simulink model "SWC_FDC_type"  (R2021b)
settings: Solver=FixedStepDiscrete  StartTime=0.0  StopTime=10.0  FixedStep=0.001  RelTol=1e-3
values from neighbouring files (symbols this model uses):
  C_TASK_5MS_S = (	C_TICK_TIME_S      	)    [vcu_local_hdr.m]
  DID_VCUKey = uint16(0x0202)    [vcu_local_hdr.m]
  DID_XWD = uint16(513)    [vcu_local_hdr.m]
  DIDLen_APPPedalZP = uint16(3)    [vcu_local_hdr.m]
  DIDLen_APSFunConfig = uint16(16)    [vcu_local_hdr.m]
  DIDLen_AutoLock = uint16(1)    [vcu_local_hdr.m]
  DIDLen_AutoWipHSpdEN = uint16(1)    [vcu_local_hdr.m]
  DIDLen_DKCKey = uint16(8)    [vcu_local_hdr.m]
  DIDLen_DRLDis = uint16(1)    [vcu_local_hdr.m]
  DIDLen_DynoMode = uint16(1)    [vcu_local_hdr.m]
  DIDLen_FMHTimer = uint16(1)    [vcu_local_hdr.m]
  DIDLen_LFLowPresThre = uint16(1)    [vcu_local_hdr.m]
  DIDLen_LFSensorID = uint16(4)    [vcu_local_hdr.m]
  DIDLen_LRLowPresThre = uint16(1)    [vcu_local_hdr.m]
  DIDLen_LRSensorID = uint16(4)    [vcu_local_hdr.m]
  DIDLen_NVMPedalZP = uint16(3)    [vcu_local_hdr.m]
  DIDLen_RFLowPresThre = uint16(1)    [vcu_local_hdr.m]
  DIDLen_RFSensorID = uint16(4)    [vcu_local_hdr.m]
  DIDLen_RRLowPresThre = uint16(1)    [vcu_local_hdr.m]
  DIDLen_RRSensorID = uint16(4)    [vcu_local_hdr.m]
  DIDLen_SensorMode = uint16(1)    [vcu_local_hdr.m]
  DIDLen_TireSize = uint16(16)    [vcu_local_hdr.m]
  DIDLen_TPMSLearnSta = uint16(1)    [vcu_local_hdr.m]
  DIDLen_TurnLampFLThreCurr = uint16(1)    [vcu_local_hdr.m]
  DIDLen_TurnLampFRThreCurr = uint16(1)    [vcu_local_hdr.m]
  DIDLen_TurnLampRLThreCurr = uint16(1)    [vcu_local_hdr.m]
  DIDLen_TurnLampRRThreCurr = uint16(1)    [vcu_local_hdr.m]
  DIDLen_USSConfig = uint16(16)    [vcu_local_hdr.m]
  DIDLen_WhlPres = uint16(4)    [vcu_local_hdr.m]
  DIDLen_WhlSensorBattSta = uint16(1)    [vcu_local_hdr.m]
  DIDLen_WhlTmp = uint16(4)    [vcu_local_hdr.m]
  DIDLen_WipRLSCmdCutFilter = uint16(1)    [vcu_local_hdr.m]
  DIDLen_WipRLSCmdHoldFilter = uint16(1)    [vcu_local_hdr.m]
  DIDLen_XWDMode = uint16(1)    [vcu_local_hdr.m]
  DIDNum_APPPedalZP = uint16(0x0206)    [vcu_local_hdr.m]
  DIDNum_APSFunConfig = uint16(0x0903)    [vcu_local_hdr.m]
  DIDNum_AutoLock = uint16(0x0306)    [vcu_local_hdr.m]
  DIDNum_AutoWipHSpdEN = uint16(0x0308)    [vcu_local_hdr.m]
  DIDNum_DKCKey = uint16(0x0202)    [vcu_local_hdr.m]
  DIDNum_DRLDis = uint16(0x0307)    [vcu_local_hdr.m]
  DIDNum_DynoMode = uint16(0x0203)    [vcu_local_hdr.m]
  DIDNum_FMHTimer = uint16(0x0305)    [vcu_local_hdr.m]
  DIDNum_LFLowPresThre = uint16(0x0B08)    [vcu_local_hdr.m]
  DIDNum_LFSensorID = uint16(0x0B01)    [vcu_local_hdr.m]
  DIDNum_LRLowPresThre = uint16(0x0B0A)    [vcu_local_hdr.m]
  DIDNum_LRSensorID = uint16(0x0B03)    [vcu_local_hdr.m]
  DIDNum_NVMPedalZP = uint16(0x0207)    [vcu_local_hdr.m]
  DIDNum_RFLowPresThre = uint16(0x0B09)    [vcu_local_hdr.m]
  DIDNum_RFSensorID = uint16(0x0B02)    [vcu_local_hdr.m]
  DIDNum_RRLowPresThre = uint16(0x0B0B)    [vcu_local_hdr.m]
  DIDNum_RRSensorID = uint16(0x0B04)    [vcu_local_hdr.m]
  DIDNum_SensorMode = uint16(0x0B0C)    [vcu_local_hdr.m]
  DIDNum_TireSize = uint16(0x0902)    [vcu_local_hdr.m]
  DIDNum_TPMSLearnSta = uint16(0x0B0D)    [vcu_local_hdr.m]
  DIDNum_TurnLampFLThreCurr = uint16(0x0303)    [vcu_local_hdr.m]
  DIDNum_TurnLampFRThreCurr = uint16(0x0301)    [vcu_local_hdr.m]
  DIDNum_TurnLampRLThreCurr = uint16(0x0304)    [vcu_local_hdr.m]
  DIDNum_TurnLampRRThreCurr = uint16(0x0302)    [vcu_local_hdr.m]
  DIDNum_USSConfig = uint16(0x0901)    [vcu_local_hdr.m]
  DIDNum_WhlPres = uint16(0x0B05)    [vcu_local_hdr.m]
  DIDNum_WhlSensorBattSta = uint16(0x0B07)    [vcu_local_hdr.m]
  DIDNum_WhlTmp = uint16(0x0B06)    [vcu_local_hdr.m]
  DIDNum_WipRLSCmdCutFilter = uint16(0x030A)    [vcu_local_hdr.m]
  DIDNum_WipRLSCmdHoldFilter = uint16(0x0309)    [vcu_local_hdr.m]
  DIDNum_XWDMode = uint16(0x0201)    [vcu_local_hdr.m]
  DIDVCUKeyLength = uint16(8)    [vcu_local_hdr.m]
  DTC_10020B = Simulink.Parameter    [DTC_Constant_Definition.m]
  DTC_10020C = Simulink.Parameter    [DTC_Constant_Definition.m]
  DTC_10020D = Simulink.Parameter    [DTC_Constant_Definition.m]
  DTC_10020E = Simulink.Parameter    [DTC_Constant_Definition.m]
  DTC_100210 = Simulink.Parameter    [DTC_Constant_Definition.m]
  DTC_100211 = Simulink.Parameter    [DTC_Constant_Definition.m]
  DTC_100212 = Simulink.Parameter    [DTC_Constant_Definition.m]
  DTC_100213 = Simulink.Parameter    [DTC_Constant_Definition.m]
  DTC_100214 = Simulink.Parameter    [DTC_Constant_Definition.m]
  DTC_100215 = Simulink.Parameter    [DTC_Constant_Definition.m]
  DTC_100216 = Simulink.Parameter    [DTC_Constant_Definition.m]
  DTC_100217 = Simulink.Parameter    [DTC_Constant_Definition.m]
  DTC_100218 = Simulink.Parameter    [DTC_Constant_Definition.m]
  DTC_100219 = Simulink.Parameter    [DTC_Constant_Definition.m]
  DTC_10021A = Simulink.Parameter    [DTC_Constant_Definition.m]
  DTC_10021B = Simulink.Parameter    [DTC_Constant_Definition.m]
  DTC_10021C = Simulink.Parameter    [DTC_Constant_Definition.m]
  DTC_10021D = Simulink.Parameter    [DTC_Constant_Definition.m]
  DTC_10021E = Simulink.Parameter    [DTC_Constant_Definition.m]
  DTC_100220 = Simulink.Parameter    [DTC_Constant_Definition.m]
  DTC_100221 = Simulink.Parameter    [DTC_Constant_Definition.m]
  DTC_100223 = Simulink.Parameter    [DTC_Constant_Definition.m]
  DTC_100224 = Simulink.Parameter    [DTC_Constant_Definition.m]
  DTC_100225 = Simulink.Parameter    [DTC_Constant_Definition.m]
  DTC_100226 = Simulink.Parameter    [DTC_Constant_Definition.m]
  DTC_100227 = Simulink.Parameter    [DTC_Constant_Definition.m]
  DTC_100242 = Simulink.Parameter    [DTC_Constant_Definition.m]
  DTC_100243 = Simulink.Parameter    [DTC_Constant_Definition.m]
  DTC_100244 = Simulink.Parameter    [DTC_Constant_Definition.m]
  DTC_100247 = Simulink.Parameter    [DTC_Constant_Definition.m]
  DTC_100248 = Simulink.Parameter    [DTC_Constant_Definition.m]
  DTC_100249 = Simulink.Parameter    [DTC_Constant_Definition.m]
  DTC_100250 = Simulink.Parameter    [DTC_Constant_Definition.m]
  DTC_100251 = Simulink.Parameter    [DTC_Constant_Definition.m]
  DTC_100252 = Simulink.Parameter    [DTC_Constant_Definition.m]
  DTC_100A10 = Simulink.Parameter    [DTC_Constant_Definition.m]
  DTC_100A12 = Simulink.Parameter    [DTC_Constant_Definition.m]
  DTC_100A16 = Simulink.Parameter    [DTC_Constant_Definition.m]
  DTC_100A17 = Simulink.Parameter    [DTC_Constant_Definition.m]
  DTC_100A18 = Simulink.Parameter    [DTC_Constant_Definition.m]
  DTC_100A19 = Simulink.Parameter    [DTC_Constant_Definition.m]
  DTC_500B01 = Simulink.Parameter    [DTC_Constant_Definition.m]
  DTC_500B02 = Simulink.Parameter    [DTC_Constant_Definition.m]
  DTC_500B03 = Simulink.Parameter    [DTC_Constant_Definition.m]
  DTC_500B04 = Simulink.Parameter    [DTC_Constant_Definition.m]
  DTC_500B05 = Simulink.Parameter    [DTC_Constant_Definition.m]
  DTC_500B06 = Simulink.Parameter    [DTC_Constant_Definition.m]
  DTC_500B07 = Simulink.Parameter    [DTC_Constant_Definition.m]
  DTC_500B08 = Simulink.Parameter    [DTC_Constant_Definition.m]
  DTC_500B09 = Simulink.Parameter    [DTC_Constant_Definition.m]
  DTC_500B0A = Simulink.Parameter    [DTC_Constant_Definition.m]
  DTC_500B0B = Simulink.Parameter    [DTC_Constant_Definition.m]
  DTC_500B0C = Simulink.Parameter    [DTC_Constant_Definition.m]
  DTC_500B0D = Simulink.Parameter    [DTC_Constant_Definition.m]
  ... (+93 more)
undefined symbols (not defined in the file or in its folder): f32_ApsOutVehSpdSig, KHAL_CANBusOffDebounce_cnt, KHAL_CANBusOffDebounce_s, KHAL_DKCDecryptEnable_flg_ovrdflg, KHAL_DKCDecryptEnable_flg_ovrdval, KHAL_RandomNumberY1_enum, KHAL_RandomNumberY2_enum, KHAL_RandomNumberY_ovrdflg, KHAL_TPMSRESBUTT_flg_ovrdflg, KHAL_TPMSRESBUTT_flg_ovrdval, KINP_ReadVinCode_flg, KTQD_DefaultRegenMode_enum, R_DIDWriteCDD_CSOP_DIDSet_APPPedalZP, R_DIDWriteCDD_CSOP_DIDSet_APSFunConfig, R_DIDWriteCDD_CSOP_DIDSet_AutoLock, R_DIDWriteCDD_CSOP_DIDSet_AutoWipHSpdEN, R_DIDWriteCDD_CSOP_DIDSet_DKCKey, R_DIDWriteCDD_CSOP_DIDSet_DRLDis, R_DIDWriteCDD_CSOP_DIDSet_DynoMode, R_DIDWriteCDD_CSOP_DIDSet_FMHTimer, R_DIDWriteCDD_CSOP_DIDSet_LFLowPresThre, R_DIDWriteCDD_CSOP_DIDSet_LFSensorID, R_DIDWriteCDD_CSOP_DIDSet_LRLowPresThre, R_DIDWriteCDD_CSOP_DIDSet_LRSensorID, R_DIDWriteCDD_CSOP_DIDSet_NVMPedalZP, R_DIDWriteCDD_CSOP_DIDSet_RFLowPresThre, R_DIDWriteCDD_CSOP_DIDSet_RFSensorID, R_DIDWriteCDD_CSOP_DIDSet_RRLowPresThre, R_DIDWriteCDD_CSOP_DIDSet_RRSensorID, R_DIDWriteCDD_CSOP_DIDSet_SensorMode, R_DIDWriteCDD_CSOP_DIDSet_TireSize, R_DIDWriteCDD_CSOP_DIDSet_TPMSLearnSta, R_DIDWriteCDD_CSOP_DIDSet_TurnLampFLThreCurr, R_DIDWriteCDD_CSOP_DIDSet_TurnLampFRThreCurr, R_DIDWriteCDD_CSOP_DIDSet_TurnLampRLThreCurr, R_DIDWriteCDD_CSOP_DIDSet_TurnLampRRThreCurr, R_DIDWriteCDD_CSOP_DIDSet_USSConfig, R_DIDWriteCDD_CSOP_DIDSet_WhlPres, R_DIDWriteCDD_CSOP_DIDSet_WhlSensorBattSta, R_DIDWriteCDD_CSOP_DIDSet_WhlTmp, R_DIDWriteCDD_CSOP_DIDSet_WipRLSCmdCutFilter, R_DIDWriteCDD_CSOP_DIDSet_WipRLSCmdHoldFilter, R_DIDWriteCDD_CSOP_DIDSet_XWDMode, R_E2E_CAN3_VCU1_CSOP_Write_CAN3_VCU1, R_E2E_CAN3_VCU1_toNIDEC_CSOP_Write_CAN3_VCU1_toNIDEC ... (+128)
libraries: simulink x246, FVT_lib x139, hcu_lib x31, hdlsllib x11, app x1, halin x1, halout x1, matrix_library x1, inp x1, outp x1
(part 4 of 13)

== system SWC_FDC_type/run_SWC_FDC_RxTx_5ms_sys/HALOUT_AFTER ==
  E2E_CAN3_VCU1_Trigger : Inport
  E2E_CAN3_VCU1_Trigger_toNIDEC : Inport  Port=2
  E2E_CAN4_VCU1_Trigger : Inport  Port=3
  function : TriggerPort  TriggerType=function-call  VariantControl=(inherit)  PortDimensions=1
  R_E2E_CAN3_VCU1_CSOP_Write_CAN3_VCU1 : Subsystem
  R_E2E_CAN3_VCU1_toNIDEC_CSOP_Write_CAN3_VCU1_toNIDEC : Subsystem
  R_E2E_CAN4_VCU1_CSOP_Write_CAN4_VCU1 : Subsystem
  wires:
  E2E_CAN3_VCU1_Trigger/1 -> R_E2E_CAN3_VCU1_CSOP_Write_CAN3_VCU1/Enable
  E2E_CAN3_VCU1_Trigger_toNIDEC/1 -> R_E2E_CAN3_VCU1_toNIDEC_CSOP_Write_CAN3_VCU1_toNIDEC/Enable
  E2E_CAN4_VCU1_Trigger/1 -> R_E2E_CAN4_VCU1_CSOP_Write_CAN4_VCU1/Enable

== system SWC_FDC_type/run_SWC_FDC_RxTx_5ms_sys/Halin_CDD ==
  PASDistanceData : Inport
  APSDistanceData : Inport  Port=2
  APSLevelData : Inport  Port=3
  APSFaultStaData : Inport  Port=4
  ChimeIn : Inport  Port=5
  SNSRLayoutIn : Inport  Port=6
  StaFSyaIn : Inport  Port=7
  ModOperationIn : Inport  Port=8
  VHAL_AccelPedal1Vol_Raw : Inport  Port=9
  VHAL_AccelPedal2Vol_Raw : Inport  Port=10
  VHAL_BrakeSWGPIO_flg : Inport  Port=11
  VHAL_HoodSW_flg : Inport  Port=12
  VHAL_TailgateSW_flg : Inport  Port=13
  VHAL_DrDoorSW_flg : Inport  Port=14
  VHAL_PsDoorSW_flg : Inport  Port=15
  VHAL_RRDoorSW_flg : Inport  Port=16
  VHAL_RLDoorSW_flg : Inport  Port=17
  VHAL_CentralDoorLockSW_flg : Inport  Port=18
  VHAL_HazardSW_flg : Inport  Port=19
  VHAL_BrakeLampSW_flg : Inport  Port=20
  VHAL_TrunkHanSW_flg : Inport  Port=21
  VHAL_SeatSW_flg : Inport  Port=22
  VHAL_CrashSignalGPIO_flg : Inport  Port=23
  u8_HWID_4byte : Inport  Port=24
  u8_GetHWIDSta : Inport  Port=25
  GetSWID_status : Inport  Port=26
  GetSWID_data : Inport  Port=27
  VHAL_AnyNMID_flg : Inport  Port=28
  VHAL_CurrentNmState_enum : Inport  Port=29
  VHAL_PwrReq_OTA_enum : Inport  Port=30
  VHAL_AllowMovThd_OTA_enum : Inport  Port=31
  VHAL_EvccAplusPwrUpReq_flg : Inport  Port=32
  VHAL_AcoreReadyToSlp_flg : Inport  Port=33
  VHAL_DidXWDSta_flg : Inport  Port=34
  VHAL_DidXWDData_enum : Inport  Port=35
  HAL_NvmReadData_raw : Inport  Port=36
  VHAL_DIDVCUKeyReadSta_flg : Inport  Port=37
  VHAL_GetDIDVCUKey_enum : Inport  Port=38
  TPMS_DataIn_flg : Inport  Port=39
  TPMS_RawData : Inport  Port=40
  BHAL_CAN2_outputs : Inport  Port=41
  BHAL_CAN4_outputs : Inport  Port=42
  VHAL_ClearDTCcmd_flg : Inport  Port=43
  VHAL_IMUOffsetVal_raw : Inport  Port=44
  VHAL_IMUSixAxisVal_raw : Inport  Port=45
  VHAL_IMUOffsetValSta_flg : Inport  Port=46
  VHAL_IMUSixAxisValSta_flg : Inport  Port=47
  VHAL_NvmProtectSta_flg : Inport  Port=48
  VHAL_AuxBattVolmV_100mV : Inport  Port=49
  VHAL_Pedal1Ref5V_raw : Inport  Port=50
  VHAL_Pedal2Ref5V_raw : Inport  Port=51
  VHAL_NetworkReqCalled_flg : Inport  Port=52
  VHAL_PmicBootReason_enum : Inport  Port=53
  VHAL_WisrBootReason_raw32 : Inport  Port=54
  BHAL_DIDGetData_raw : Inport  Port=55
  VHAL_AcoreRebootCmd_raw : Inport  Port=56
  VHAL_CAN1BusOff_raw : Inport  Port=57
  VHAL_CAN2BusOff_raw : Inport  Port=58
  VHAL_CAN3BusOff_raw : Inport  Port=59
  VHAL_CAN4BusOff_raw : Inport  Port=60
  VHAL_CAN5BusOff_raw : Inport  Port=61
  VHAL_CAN6BusOff_raw : Inport  Port=62
  u8_GetAPS_Progress_PCT : Inport  Port=63
  u8_GetAPS_RQ_Display : Inport  Port=64
  u8_GetAPS_SW_Ver : Inport  Port=65
  u8_GetAPS_HW_Ver : Inport  Port=66
  u8_GetAPS_ExitCondition : Inport  Port=67
  f32_GetAPS_Angle_Target : Inport  Port=68
  u8_GetAPS_Sta_System : Inport  Port=69
  u8_GetAPS_V_Rq_EPAS_Ctrl : Inport  Port=70
  u8_GetAPS_Rq_EPAS_Ctrl : Inport  Port=71
  u8_GetAPS_Req : Inport  Port=72
  f32_GetAPS_DecReq : Inport  Port=73
  u8_GetAPS_DecReq_A : Inport  Port=74
  f32_GetAPS_SpeedCmd : Inport  Port=75
  u8_GetAPS_ShftPosnReq : Inport  Port=76
  u8_GetAPS_VMC_Req_A : Inport  Port=77
  u8_GetCAAS_Sta : Inport  Port=78
  u8_GetCAAS_VMC_Req_A : Inport  Port=79
  u8_TPMSSensorIDRegSta : Inport  Port=80
  u8_ResetPedalZeroPosReq : Inport  Port=81
  u8_GetAPS_PwrReq_cmd : Inport  Port=82
  u8_GetRAPS_BCM_LockReq_Cmd : Inport  Port=83
  u8_GetRAPS_BCM_Lamp_Cmd : Inport  Port=84
  u8_GetRAPS_ErrWarn_Sta : Inport  Port=85
  u8_GetRAPS_ErrLv1_flg : Inport  Port=86
  u32_BootPath : Inport  Port=87
  VHAL_CAN1RxErrorCount_raw : Inport  Port=88
  VHAL_CAN1TxErrorCount_raw : Inport  Port=89
  VHAL_CAN2RxErrorCount_raw : Inport  Port=90
  VHAL_CAN2TxErrorCount_raw : Inport  Port=91
  VHAL_CAN3RxErrorCount_cnt : Inport  Port=92
  VHAL_CAN3TxErrorCount_raw : Inport  Port=93
  VHAL_CAN4RxErrorCount_raw : Inport  Port=94
  VHAL_CAN4TxErrorCount_raw : Inport  Port=95
  VHAL_CAN5RxErrorCount_raw : Inport  Port=96
  VHAL_CAN5TxErrorCount_raw : Inport  Port=97
  VHAL_CAN6RxErrorCount_raw : Inport  Port=98
  VHAL_CAN6TxErrorCount_raw : Inport  Port=99
  trig_HalinCDD : TriggerPort  TriggerType=function-call  VariantControl=(inherit)
  Halin_APM : Subsystem
  Halin_DKC_A : Subsystem
  Halin_GPIO : Subsystem
  Halin_IMU : Subsystem
  Halin_SYS : Subsystem
  Halin_TPMS : Subsystem
  Subsystem : Subsystem
  TPM_Scheduler : Stateflow chart  TreatAsAtomicUnit=on
  BHAL_APM_outputs : Outport
  BHAL_GPIO_outputs : Outport  Port=2
  BHAL_SYS_outputs : Outport  Port=3
  BHAL_TPMS_outputs : Outport  Port=4
  BHAL_SYSTPMS_outputs : Outport  Port=5
  BHAL_DDM_outputs : Outport  Port=6
  BHAL_IMU_outputs : Outport  Port=7
  Enable_decrypt : Outport  Port=8
  AESKey : Outport  Port=9
  DKCRawData : Outport  Port=10
  wires:
  Halin_DKC_A/1(Enable_Decrypt) -> Enable_decrypt/1
  VHAL_RLDoorSW_flg/1 -> Halin_GPIO/9(VHAL_RLDoorSW_flg)
  Halin_SYS/1(BHAL_SYS_outputs) -> [BHAL_SYS_outputs], BHAL_SYS_outputs/1
  Halin_DKC_A/3(DKCRawData) -> DKCRawData/1
  GetSWID_data/1 -> Halin_SYS/2(GetSWID_data)
  VHAL_GetDIDVCUKey_enum/1 -> Halin_SYS/13(VHAL_GetDIDVCUKey_enum)
  VHAL_TailgateSW_flg/1 -> Halin_GPIO/5(VHAL_TailgateSW_flg)
  Halin_DKC_A/2(AESKey) -> AESKey/1
  VHAL_AccelPedal2Vol_Raw/1 -> Halin_GPIO/2(VHAL_AccelPedal2Vol_Raw)
  TPM_Scheduler/1(trig_TPM_10ms1()) -> Halin_TPMS/Trigger
  VHAL_TrunkHanSW_flg/1 -> Halin_GPIO/13(VHAL_TrunkHanSW_flg)
  VHAL_DidXWDSta_flg/1 -> Halin_SYS/9(VHAL_DidXWDSta_flg)
  VHAL_CurrentNmState_enum/1 -> Halin_SYS/4(VHAL_CurrentNmState_enum)
  VHAL_AccelPedal1Vol_Raw/1 -> Halin_GPIO/1(VHAL_AccelPedal1Vol_Raw)
  u8_HWID_4byte/1 -> Halin_GPIO/16(u8_HWID_4byte)
  BHAL_CAN2_outputs/1 -> Halin_TPMS/3(BHAL_CAN2_outputs)
  VHAL_AcoreReadyToSlp_flg/1 -> Halin_SYS/8(VHAL_AcoreReadyToSlp_flg)
  HAL_NvmReadData_raw/1 -> Halin_SYS/11(HAL_NvmReadData_raw)
  VHAL_AllowMovThd_OTA_enum/1 -> Halin_SYS/6(VHAL_AllowMovThd_OTA_enum)
  VHAL_BrakeLampSW_flg/1 -> Halin_GPIO/12(VHAL_BrakeLampSW_flg)
  VHAL_RRDoorSW_flg/1 -> Halin_GPIO/8(VHAL_RRDoorSW_flg)
  VHAL_BrakeSWGPIO_flg/1 -> Halin_GPIO/3(VHAL_BrakeSWGPIO_flg)
  GetSWID_status/1 -> Halin_SYS/1(GetSWID_status)
  VHAL_DrDoorSW_flg/1 -> Halin_GPIO/6(VHAL_DrDoorSW_flg)
  VHAL_PwrReq_OTA_enum/1 -> Halin_SYS/5(VHAL_PwrReq_OTA_enum)
  VHAL_HoodSW_flg/1 -> Halin_GPIO/4(VHAL_HoodSW_flg)
  Halin_GPIO/1(BHAL_GPIO_outputs) -> BHAL_GPIO_outputs/1
  BHAL_CAN4_outputs/1 -> Halin_DKC_A/1(BHAL_CAN4_outputs)
  VHAL_CentralDoorLockSW_flg/1 -> Halin_GPIO/10(VHAL_CentralDoorLockSW_flg)
  TPMS_RawData/1 -> Halin_TPMS/2(TPMS_RawData)
  VHAL_CrashSignalGPIO_flg/1 -> Halin_GPIO/15(VHAL_CrashSignalGPIO_flg)
  Halin_TPMS/1(BHAL_TPMS_outputs) -> BHAL_TPMS_outputs/1
  VHAL_DidXWDData_enum/1 -> Halin_SYS/10(VHAL_DidXWDData_enum)
  VHAL_EvccAplusPwrUpReq_flg/1 -> Halin_SYS/7(VHAL_EvccAplusPwrUpReq_flg)
  VHAL_SeatSW_flg/1 -> Halin_GPIO/14(VHAL_SeatSW_flg)
  VHAL_DIDVCUKeyReadSta_flg/1 -> Halin_SYS/12(VHAL_DIDVCUKeyReadSta_flg)
  VHAL_PsDoorSW_flg/1 -> Halin_GPIO/7(VHAL_PsDoorSW_flg)
  [BHAL_SYS_outputs] -> Halin_DKC_A/2(BHAL_SYS_outputs)
  TPMS_DataIn_flg/1 -> Halin_TPMS/1(TPMS_DataIn_flg)
  VHAL_AnyNMID_flg/1 -> Halin_SYS/3(VHAL_AnyNMID_flg)
  VHAL_HazardSW_flg/1 -> Halin_GPIO/11(VHAL_HazardSW_flg)
  Halin_SYS/2(BHAL_SYSTPMS_outputs) -> [BHAL_SYSTPMS_outputs], BHAL_SYSTPMS_outputs/1
  [BHAL_SYSTPMS_outputs] -> Halin_TPMS/4(BHAL_SYSTPMS_outputs)
  VHAL_ClearDTCcmd_flg/1 -> Subsystem/1(VHAL_ClearDTCcmd_flg)
  Subsystem/1(BHAL_DDM_outputs) -> BHAL_DDM_outputs/1
  Halin_IMU/1(BHAL_IMU_outputs) -> BHAL_IMU_outputs/1
  VHAL_IMUOffsetVal_raw/1 -> Halin_IMU/1(VHAL_IMUOffsetVal_raw)
  VHAL_IMUOffsetValSta_flg/1 -> Halin_IMU/3(VHAL_IMUOffsetValSta_flg)
  VHAL_IMUSixAxisVal_raw/1 -> Halin_IMU/2(VHAL_IMUSixAxisVal_raw)
  VHAL_IMUSixAxisValSta_flg/1 -> Halin_IMU/4(VHAL_IMUSixAxisValSta_flg)
  VHAL_NvmProtectSta_flg/1 -> Halin_SYS/14(VHAL_NvmProtectSta_flg)
  VHAL_AuxBattVolmV_100mV/1 -> Halin_SYS/15(VHAL_AuxBattVolmV_100mV)
  VHAL_Pedal1Ref5V_raw/1 -> Halin_SYS/16(VHAL_Pedal1Ref5V_raw)
  VHAL_Pedal2Ref5V_raw/1 -> Halin_SYS/17(VHAL_Pedal2Ref5V_raw)
  VHAL_NetworkReqCalled_flg/1 -> Halin_SYS/18(VHAL_NetworkReqCalled_flg)
  VHAL_PmicBootReason_enum/1 -> Halin_SYS/19(VHAL_PmicBootReason_enum)
  VHAL_WisrBootReason_raw32/1 -> Halin_SYS/20(VHAL_WisrBootReason_raw32)
  BHAL_DIDGetData_raw/1 -> Halin_SYS/21(BHAL_DIDGetData_raw)
  VHAL_AcoreRebootCmd_raw/1 -> Halin_SYS/22(VHAL_AcoreRebootCmd_raw)
  VHAL_CAN1BusOff_raw/1 -> Halin_SYS/23(VHAL_CAN1BusOff_raw)
  VHAL_CAN2BusOff_raw/1 -> Halin_SYS/24(VHAL_CAN2BusOff_raw)
  VHAL_CAN3BusOff_raw/1 -> Halin_SYS/25(VHAL_CAN3BusOff_raw)
  VHAL_CAN4BusOff_raw/1 -> Halin_SYS/26(VHAL_CAN4BusOff_raw)
  VHAL_CAN5BusOff_raw/1 -> Halin_SYS/27(VHAL_CAN5BusOff_raw)
  Halin_APM/1(BHAL_APM_outputs) -> BHAL_APM_outputs/1
  u8_TPMSSensorIDRegSta/1 -> Halin_SYS/29(VHAL_TPMSSensorIDRegSta_raw)
  u8_ResetPedalZeroPosReq/1 -> Halin_SYS/30(VHAL_ResetPedalZeroPosReq_raw)
  u8_GetHWIDSta/1 -> Halin_GPIO/17(u8_GetHWIDSta)
  PASDistanceData/1 -> Halin_APM/1(PASDistanceData)
  APSDistanceData/1 -> Halin_APM/2(APSDistanceData)
  APSLevelData/1 -> Halin_APM/3(APSLevelData)
  APSFaultStaData/1 -> Halin_APM/4(APSFaultStaData)
  ChimeIn/1 -> Halin_APM/5(ChimeIn)
  SNSRLayoutIn/1 -> Halin_APM/6(SNSRLayoutIn)
  StaFSyaIn/1 -> Halin_APM/7(StaFSyaIn)
  ModOperationIn/1 -> Halin_APM/8(ModOperationIn)
  u8_GetAPS_Progress_PCT/1 -> Halin_APM/9(u8_GetAPS_Progress_PCT)
  u8_GetAPS_RQ_Display/1 -> Halin_APM/10(u8_GetAPS_RQ_Display)
  u8_GetAPS_SW_Ver/1 -> Halin_APM/11(u8_GetAPS_SW_Ver)
  u8_GetAPS_HW_Ver/1 -> Halin_APM/12(u8_GetAPS_HW_Ver)
  u8_GetAPS_ExitCondition/1 -> Halin_APM/13(u8_GetAPS_ExitCondition)
  f32_GetAPS_Angle_Target/1 -> Halin_APM/14(f32_GetAPS_Angle_Target)
  u8_GetAPS_Sta_System/1 -> Halin_APM/15(u8_GetAPS_Sta_System)
  u8_GetAPS_V_Rq_EPAS_Ctrl/1 -> Halin_APM/16(u8_GetAPS_V_Rq_EPAS_Ctrl)
  u8_GetAPS_Rq_EPAS_Ctrl/1 -> Halin_APM/17(u8_GetAPS_Rq_EPAS_Ctrl)
  u8_GetAPS_Req/1 -> Halin_APM/18(u8_GetAPS_Req)
  f32_GetAPS_DecReq/1 -> Halin_APM/19(f32_GetAPS_DecReq)
  u8_GetAPS_DecReq_A/1 -> Halin_APM/20(u8_GetAPS_DecReq_A)
  f32_GetAPS_SpeedCmd/1 -> Halin_APM/21(f32_GetAPS_SpeedCmd)
  u8_GetAPS_ShftPosnReq/1 -> Halin_APM/22(u8_GetAPS_ShftPosnReq)
  u8_GetAPS_VMC_Req_A/1 -> Halin_APM/23(u8_GetAPS_VMC_Req_A)
  u8_GetCAAS_Sta/1 -> Halin_APM/24(u8_GetCAAS_Sta)
  u8_GetCAAS_VMC_Req_A/1 -> Halin_APM/25(u8_GetCAAS_VMC_Req_A)
  u8_GetAPS_PwrReq_cmd/1 -> Halin_APM/26(u8_GetAPS_PwrReq_cmd)
  u8_GetRAPS_BCM_LockReq_Cmd/1 -> Halin_APM/27(u8_GetRAPS_BCM_LockReq_Cmd)
  u8_GetRAPS_BCM_Lamp_Cmd/1 -> Halin_APM/28(u8_GetRAPS_BCM_Lamp_Cmd)
  u8_GetRAPS_ErrWarn_Sta/1 -> Halin_APM/29(u8_GetRAPS_ErrWarn_Sta)
  u8_GetRAPS_ErrLv1_flg/1 -> Halin_APM/30(u8_GetRAPS_ErrLv1_flg)
  VHAL_CAN6BusOff_raw/1 -> Halin_SYS/28(VHAL_CAN6BusOff_raw)
  u32_BootPath/1 -> Halin_SYS/31(VHAL_PmicBootPath_raw32)
  VHAL_CAN1RxErrorCount_raw/1 -> Halin_SYS/32(VHAL_CAN1RxErrorCount_raw)
  VHAL_CAN1TxErrorCount_raw/1 -> Halin_SYS/33(VHAL_CAN1TxErrorCount_raw)
  VHAL_CAN2RxErrorCount_raw/1 -> Halin_SYS/34(VHAL_CAN2RxErrorCount_raw)
  VHAL_CAN2TxErrorCount_raw/1 -> Halin_SYS/35(VHAL_CAN2TxErrorCount_raw)
  VHAL_CAN3RxErrorCount_cnt/1 -> Halin_SYS/36(VHAL_CAN3RxErrorCount_raw)
  VHAL_CAN3TxErrorCount_raw/1 -> Halin_SYS/37(VHAL_CAN3TxErrorCount_raw)
  VHAL_CAN4RxErrorCount_raw/1 -> Halin_SYS/38(VHAL_CAN4RxErrorCount_raw)
  VHAL_CAN4TxErrorCount_raw/1 -> Halin_SYS/39(VHAL_CAN4TxErrorCount_raw)
  VHAL_CAN5RxErrorCount_raw/1 -> Halin_SYS/40(VHAL_CAN5RxErrorCount_raw)
  VHAL_CAN5TxErrorCount_raw/1 -> Halin_SYS/41(VHAL_CAN5TxErrorCount_raw)
  VHAL_CAN6RxErrorCount_raw/1 -> Halin_SYS/42(VHAL_CAN6RxErrorCount_raw)
  VHAL_CAN6TxErrorCount_raw/1 -> Halin_SYS/43(VHAL_CAN6TxErrorCount_raw)

== system SWC_FDC_type/run_SWC_FDC_RxTx_5ms_sys/OUTP_AFTER ==
  BOUTP_outputs : Inport
  BHAL_SYSTPMS_outputs : Inport  Port=2
  BHAL_SYS_outputs : Inport  Port=3
  VHAL_NvmReadArray_raw : Inport  Port=4
  BHAL_DIDGetData_raw : Inport  Port=5
  trig_OUTP_After : TriggerPort  TriggerType=function-call  VariantControl=(inherit)
  APM : Subsystem
  DID_list : Subsystem
  DTC_list : Subsystem
  Subsystem5 : Subsystem
  ApsOut_GearPosnSig : Outport
  ApsOut_SendChrgPlugStaSig : Outport  Port=2
  ApsOut_SetFrSensorOnCmd : Outport  Port=3
  ApsOut_SetFrSensorSwTOCmd : Outport  Port=4
  ApsOut_SetVehSpdTOCmd : Outport  Port=5
  ApsOut_VehSpdSig : Outport  Port=6
  HAL_NvmWriteData_raw : Outport  Port=7
  DTC_Trigger : Outport  Port=8
  Header_Array : Outport  Port=9
  DTC_Constant_Array : Outport  Port=10
  DTC_Array : Outport  Port=11
  BOUTP_DIDSetData_outputs : Outport  Port=12
  wires:
  APM/1(ApsOut_GearPosnSig) -> ApsOut_GearPosnSig/1
  Subsystem5/1(HAL_NvmWriteData_raw) -> HAL_NvmWriteData_raw/1
  APM/2(ApsOut_SendChrgPlugStaSig) -> ApsOut_SendChrgPlugStaSig/1
  APM/5(ApsOut_SetVehSpdTOCmd) -> ApsOut_SetVehSpdTOCmd/1
  APM/3(ApsOut_SetFrSensorOnCmd) -> ApsOut_SetFrSensorOnCmd/1
  BOUTP_outputs/1 -> [BOUTP_outputs]
  APM/6(ApsOut_VehSpdSig) -> ApsOut_VehSpdSig/1
  APM/4(ApsOut_SetFrSensorSwTOCmd) -> ApsOut_SetFrSensorSwTOCmd/1
  [BOUTP_outputs] -> APM/1(BOUTP_outputs)
  [BOUTP_outputs] -> Subsystem5/1(BOUTP_outputs)
  BHAL_SYSTPMS_outputs/1 -> [BHAL_SYSTPMS_outputs]
  [BHAL_SYSTPMS_outputs] -> Subsystem5/2(BHAL_SYSTPMS_outputs)
  [BOUTP_outputs] -> DTC_list/1(BOUTP_outputs)
  DTC_list/1(Trigger) -> DTC_Trigger/1
  DTC_list/2(Header_Array) -> Header_Array/1
  DTC_list/4(DTC_Array) -> DTC_Array/1
  BHAL_SYS_outputs/1 -> [BHAL_SYS_outputs]
  [BHAL_SYS_outputs] -> Subsystem5/3(BHAL_SYS_outputs)
  DID_list/1(BOUTP_DIDSetData_outputs) -> BOUTP_DIDSetData_outputs/1
  [BOUTP_outputs] -> DID_list/1(BOUTP_outputs)
  VHAL_NvmReadArray_raw/1 -> [VHAL_NvmReadArray_raw]
  [VHAL_NvmReadArray_raw] -> DID_list/2(VHAL_NvmReadArray_raw)
  BHAL_DIDGetData_raw/1 -> [BHAL_DIDGetData_raw]
  [BHAL_DIDGetData_raw] -> Subsystem5/4(BHAL_DIDGetData_raw)
  DTC_list/3(DTC_Constant_Array) -> DTC_Constant_Array/1

== system SWC_FDC_type/run_SWC_FDC_RxTx_5ms_sys/R_FDCCDD_Inner_CSOP_FDC_AppCallSleep ==
  Enable : EnablePort
  R_FDCCDD_Inner_CSOP_FDC_AppCallSleep : FunctionCaller  FunctionPrototype=R_FDCCDD_Inner_CSOP_FDC_AppCallSleep()

== system SWC_FDC_type/run_SWC_FDC_RxTx_5ms_sys/R_HALIN_IMU_CSOP_IMUGetOffsetVal ==
  trig_ReadIMUOffset_00 : TriggerPort  TriggerType=function-call  VariantControl=(inherit)  PortDimensions=1
  R_HALIN_IMU_CSOP_IMUGetOffsetVal : FunctionCaller  FunctionPrototype=[s16_IMUOffsetVal,u8_IMUOffsetValSta] = R_HALIN_IMU_CSOP_IMUGetOffsetVal()  OutputArgumentSpecifications=int16([1;1;1;1;1;1]), uint8(1)
  Out1 : Outport
  Out2 : Outport  Port=2
  wires:
  R_HALIN_IMU_CSOP_IMUGetOffsetVal/2 -> Out2/1
  R_HALIN_IMU_CSOP_IMUGetOffsetVal/1 -> Out1/1

== system SWC_FDC_type/run_SWC_FDC_RxTx_5ms_sys/R_HALIN_IMU_CSOP_IMUSetSta ==
  u8_IMUEnaCmd : Inport
  Enable : EnablePort
  R_HALIN_IMU_CSOP_IMUSetSta : FunctionCaller  FunctionPrototype=R_HALIN_IMU_CSOP_IMUSetSta(u8_IMUEnaCmd)  InputArgumentSpecifications=uint8(1)
  wires:
  u8_IMUEnaCmd/1 -> R_HALIN_IMU_CSOP_IMUSetSta/1

== system SWC_FDC_type/run_SWC_FDC_RxTx_5ms_sys/R_HALOUTCDD_CSOP_AppNmStateReq ==
  WakeReq : Inport
  SleepReq : Inport  Port=2
  Enable : EnablePort
  Latch : hcu_lib/Basic_Blocks/Latch
  R_HALOUTCDD_CSOP_AppNmStateReq : FunctionCaller  FunctionPrototype=R_HALOUTCDD_CSOP_AppNmStateReq(u8_WakeUpReq,u8_SleepReq)  InputArgumentSpecifications=uint8(1), uint8(1)
  Outport : Outport
  wires:
  SleepReq/1 -> R_HALOUTCDD_CSOP_AppNmStateReq/2
  Latch/1 -> Outport/1
  WakeReq/1 -> Latch/1, R_HALOUTCDD_CSOP_AppNmStateReq/1

== system SWC_FDC_type/run_SWC_FDC_RxTx_5ms_sys/R_HALOUTCDD_CSOP_SetAcoreRebootCmdACK ==
  Enable : EnablePort
  R_HALOUTCDD_CSOP_SetAcoreRebootCmdACK : FunctionCaller  FunctionPrototype=R_HALOUTCDD_CSOP_SetAcoreRebootCmdACK()

== system SWC_FDC_type/run_SWC_FDC_RxTx_5ms_sys/R_HALOUTCDD_CSOP_SleepRequest ==
  SleepState : Inport
  WakeUpTime : Inport  Port=2
  Enable : EnablePort
  R_HALOUTCDD_CSOP_SleepRequest : FunctionCaller  FunctionPrototype=R_HALOUTCDD_CSOP_SleepRequest(u32_SleepyState,u32_Wakeup_Timer_s)  InputArgumentSpecifications=uint32(1), uint32(1)
  wires:
  WakeUpTime/1 -> R_HALOUTCDD_CSOP_SleepRequest/2
  SleepState/1 -> R_HALOUTCDD_CSOP_SleepRequest/1

== system SWC_FDC_type/run_SWC_FDC_RxTx_5ms_sys/R_NVMReadCDD_Inner_NVM_ReadOperation ==
  trig_ReadNVM : TriggerPort  TriggerType=function-call  VariantControl=(inherit)  PortDimensions=1
  R_NVMReadCDD_Inner_NVM_ReadOperation : FunctionCaller  FunctionPrototype=R_NVMReadCDD_Inner_NVM_ReadOperation()

== system SWC_FDC_type/run_SWC_FDC_RxTx_5ms_sys/R_NVMWriteCDD_Inner_NVM_WriteOperation ==
  Enable : EnablePort
  R_NVMWriteCDD_Inner_NVM_WriteOperation : FunctionCaller  FunctionPrototype=R_NVMWriteCDD_Inner_NVM_WriteOperation()

== system SWC_FDC_type/run_SWC_FDC_RxTx_5ms_sys/R_UDSCDD_CSOP_DdmRestartOperationCycle ==
  Enable : EnablePort
  R_UDSCDD_CSOP_DdmRestartOperationCycle : FunctionCaller  FunctionPrototype=R_UDSCDD_CSOP_DdmRestartOperationCycle()

== system SWC_FDC_type/run_SWC_FDC_RxTx_5ms_sys/R_UDSCDD_CSOP_SetDTCStatus ==
  Header_Array : Inport
  DTC_Array : Inport  Port=2
  DTC_Constant_Array : Inport  Port=3
  Enable : EnablePort
  R_UDSCDD_CSOP_SetDTCStatus : FunctionCaller  FunctionPrototype=u8_ReturnStatus = R_UDSCDD_CSOP_SetDTCStatus(u32Array10_Header,u32Array320_DTC,u16Array320_DTCConst)  InputArgumentSpecifications=uint32([1;1;1;1;1;1;1;1;1;1]), uint32([1;1;1;1;1;1;1;1;1;1;1;1;1;1;1;1;1;1;1;1;1;1;1;1;1;1;1;1;1;1;1;1;1;1;1;1;1;1;1;1;1;1;1;1;1;1;1;1;1;1;1;1;1;1;1;1;1;1;1;1;1;1;1;1;1;1;1;1;1;1;1;1;1;1;1;1;1;1;1;1;1;1;1;1;1;1;1;1;1;1;1;1;1;1;1;1;1;1;1;1;1;1;1;1;1;1;1;1;1;1;1;1;1;1;1;1;1;1;1;1;1;1;1;1;1;1;1;1;1;1;1;1;1;1;1;1;1;1;1;1;1;1;1;1;1;1;1;1;1;1;1;1;1;1;1;1;1;1;1;1;1;1;1;1;1;1;1;1;1;1;1;1;1;1;1;1;1;1;1;1;1;1;1;1;1;1;1;1;1;1;1;1;1;1;1;1;1;1;1;1;1;1;1;1;1;1;1;1;1;1;1;1;1;1;1;1;1;1;1;1;1;1;1;1;1;1;1;1;1;1;1;1;1;1;1;1;1;1;1;1;1;1;1;1;1;1;1;1;1;1;1;1;1;1;1;1;1;1;1;1;1;1;1;1;1;1;1;1;1;1;1;1;1;1;1;1;1;1;1;1;1;1;1;1;1;1;1;1;1;1;1;1;1;1;1;1;1;1;1;1;1;1;1;1;1;1;1;1;1;1;1;1;1;1;1;1;1;1;1;1]), uint16([1;1;1;1;1;1;1;1;1;1;1;1;1;1;1;1;1;1;1;1;1;1;1;1;1;1;1;1;1;1;1;1;1;1;1;1;1;1;1;1;1;1;1;1;1;1;1;1;1;1;1;1;1;1;1;1;1;1;1;1;1;1;1;1;1;1;1;1;1;1;1;1;1;1;1;1;1;1;1;1;1;1;1;1;1;1;1;1;1;1;1;1;1;1;1;1;1;1;1;1;1;1;1;1;1;1;1;1;1;1;1;1;1;1;1;1;1;1;1;1;1;1;1;1;1;1;1;1;1;1;1;1;1;1;1;1;1;1;1;1;1;1;1;1;1;1;1;1;1;1;1;1;1;1;1;1;1;1;1;1;1;1;1;1;1;1;1;1;1;1;1;1;1;1;1;1;1;1;1;1;1;1;1;1;1;1;1;1;1;1;1;1;1;1;1;1;1;1;1;1;1;1;1;1;1;1;1;1;1;1;1;1;1;1;1;1;1;1;1;1;1;1;1;1;1;1;1;1;1;1;1;1;1;1;1;1;1;1;1;1;1;1;1;1;1;1;1;1;1;1;1;1;1;1;1;1;1;1;1;1;1;1;1;1;1;1;1;1;1;1;1;1;1;1;1;1;1;1;1;1;1;1;1;1;1;1;1;1;1;1;1;1;1;1;1;1;1;1;1;1;1;1;1;1;1;1;1;1;1;1;1;1;1;1;1;1;1;1;1;1])  OutputArgumentSpecifications=uint8(1)
  retSta : Outport
  wires:
  Header_Array/1 -> R_UDSCDD_CSOP_SetDTCStatus/1
  DTC_Array/1 -> R_UDSCDD_CSOP_SetDTCStatus/2
  R_UDSCDD_CSOP_SetDTCStatus/1 -> retSta/1
  DTC_Constant_Array/1 -> R_UDSCDD_CSOP_SetDTCStatus/3

== system SWC_FDC_type/run_SWC_FDC_RxTx_5ms_sys/R_WDGCDD_CSOP_Call_WDG_AppEnd ==
  Enable : EnablePort
  R_WDGCDD_CSOP_Call_WDG_AppEnd : FunctionCaller  FunctionPrototype=R_WDGCDD_CSOP_Call_WDG_AppEnd()

== system SWC_FDC_type/run_SWC_FDC_RxTx_5ms_sys/R_WDGCDD_CSOP_Call_WDG_AppStart ==
  Enable : EnablePort
  R_WDGCDD_CSOP_Call_WDG_AppStart : FunctionCaller  FunctionPrototype=R_WDGCDD_CSOP_Call_WDG_AppStart()

== system SWC_FDC_type/run_SWC_FDC_RxTx_5ms_sys/R_WDGCDD_CSOP_Call_Watchdog ==
  trig_WDG : TriggerPort  TriggerType=function-call  VariantControl=(inherit)  PortDimensions=1
  R_WDGCDD_CSOP_Call_Watchdog : FunctionCaller  FunctionPrototype=R_WDGCDD_CSOP_Call_Watchdog()

== system SWC_FDC_type/run_SWC_FDC_RxTx_5ms_sys/Subsystem ==
  In1 : Inport
  Enable : EnablePort
  R_HALINCDD_CSOP_TPMSSensorIDRegSetResults : FunctionCaller  FunctionPrototype=R_HALINCDD_CSOP_TPMSSensorIDRegSetResults(u8Array2_TPMSSensorIDRegResults)  InputArgumentSpecifications=uint8([1;1])
  wires:
  In1/1 -> R_HALINCDD_CSOP_TPMSSensorIDRegSetResults/1

== system SWC_FDC_type/run_SWC_FDC_RxTx_5ms_sys/Subsystem1 ==
  Enable : EnablePort
  R_HALINCDD_CSOP_ResetPedalZeroPosDone : FunctionCaller  FunctionPrototype=R_HALINCDD_CSOP_ResetPedalZeroPosDone()

== system SWC_FDC_type/run_SWC_FDC_RxTx_5ms_sys/Subsystem2 ==
  VHAL_DIDSetNVMPedalZP_raw8 : Inport
  Enable : EnablePort
  DIDLen7 : Constant  Value=DIDNum_NVMPedalZP
  DIDNum7 : Constant  Value=DIDLen_NVMPedalZP
  R_DIDWriteCDD_CSOP_DIDSet_NVMPedalZP : FunctionCaller  FunctionPrototype=R_DIDWriteCDD_CSOP_DIDSet_NVMPedalZP(u16_DIDNum_NVMPedalZP,u16_DIDLen_NVMPedalZP,u8Array3_NVMPedalZP)  InputArgumentSpecifications=uint16(1), uint16(1), uint8([1;1;1])
  wires:
  DIDLen7/1 -> R_DIDWriteCDD_CSOP_DIDSet_NVMPedalZP/1
  VHAL_DIDSetNVMPedalZP_raw8/1 -> R_DIDWriteCDD_CSOP_DIDSet_NVMPedalZP/3
  DIDNum7/1 -> R_DIDWriteCDD_CSOP_DIDSet_NVMPedalZP/2

== system SWC_FDC_type/run_SWC_FDC_RxTx_5ms_sys/Subsystem3 ==
  AESKey : Inport
  DKCRawData : Inport  Port=2
  function : TriggerPort  TriggerType=function-call  VariantControl=(inherit)
  R_HALINCDD_CSOP_DKCDecrypt : FunctionCaller  FunctionPrototype=u8Array16_ResultData = R_HALINCDD_CSOP_DKCDecrypt(u8Array16_AESkey,u8Array16_RawData)  InputArgumentSpecifications=uint8([1;1;1;1;1;1;1;1;1;1;1;1;1;1;1;1]), uint8([1;1;1;1;1;1;1;1;1;1;1;1;1;1;1;1])  OutputArgumentSpecifications=uint8([1;1;1;1;1;1;1;1;1;1;1;1;1;1;1;1])
  u8Array16_ResultData : Outport
  wires:
  R_HALINCDD_CSOP_DKCDecrypt/1 -> u8Array16_ResultData/1
  AESKey/1 -> R_HALINCDD_CSOP_DKCDecrypt/1
  DKCRawData/1 -> R_HALINCDD_CSOP_DKCDecrypt/2

== system SWC_FDC_type/run_SWC_FDC_RxTx_5ms_sys/Subsystem4 ==
  Enable_Decrypt : Inport
  u8Array16_ResultData : Inport  Port=2
  function : TriggerPort  TriggerType=function-call  VariantControl=(inherit)
  DKC2 : Subsystem  AncestorBlock=halin_NA_Ref/HAL_IN/DKC1
  Data Type Conversion97 : DataTypeConversion  OutDataTypeStr=uint8
  BHAL_DKC_outputs : Outport
  wires:
  [u8Array16_ResultData] -> Data Type Conversion97/1
  DKC2/1(BHAL_DKC_outputs) -> BHAL_DKC_outputs/1
  Data Type Conversion97/1 -> DKC2/2(DKC_ResultData_16byte)
  Enable_Decrypt/1 -> DKC2/1(Enable_Decrypt)
  u8Array16_ResultData/1 -> [u8Array16_ResultData]

== system SWC_FDC_type/run_SWC_FDC_RxTx_5ms_sys/Subsystem5 ==
  In1 : Inport
  Enable : EnablePort
  R_HALOUTCDD_CSOP_IVIReset : FunctionCaller  FunctionPrototype=R_HALOUTCDD_CSOP_IVIReset(u8_RstValue)  InputArgumentSpecifications=uint8(1)
  wires:
  In1/1 -> R_HALOUTCDD_CSOP_IVIReset/1

== system SWC_FDC_type/run_SWC_FDC_RxTx_5ms_sys/Subsystem6 ==
  Enable : EnablePort
  R_HALINCDD_CSOP_GetVinCode : FunctionCaller  FunctionPrototype=u8Array17_VinCode = R_HALINCDD_CSOP_GetVinCode()  OutputArgumentSpecifications=uint8([1;1;1;1;1;1;1;1;1;1;1;1;1;1;1;1;1])
  u8Array17_VinCode : Outport
  wires:
  R_HALINCDD_CSOP_GetVinCode/1 -> u8Array17_VinCode/1

== system SWC_FDC_type/run_SWC_FDC_RxTx_5ms_sys/Subsystem7 ==
  u8Array17_VinCode : Inport
  Data Type Conversion{,1..16} (17 alike) : DataTypeConversion
  Demux : Demux  Outputs=17
  Display{1..17} (17 alike) : Display
  wires:
  Demux/1 -> Data Type Conversion/1
  u8Array17_VinCode/1 -> Demux/1
  Data Type Conversion/1 -> Display1/1  "VINP_VinCodeByte0_enum"
  Data Type Conversion1/1 -> Display2/1  "VINP_VinCodeByte1_enum"
  Demux/2 -> Data Type Conversion1/1
  Demux/3 -> Data Type Conversion2/1
  Demux/4 -> Data Type Conversion3/1
  Demux/5 -> Data Type Conversion4/1
  Demux/6 -> Data Type Conversion5/1
  Demux/7 -> Data Type Conversion6/1
  Data Type Conversion2/1 -> Display3/1  "VINP_VinCodeByte2_enum"
  Data Type Conversion3/1 -> Display4/1  "VINP_VinCodeByte3_enum"
  Data Type Conversion4/1 -> Display5/1  "VINP_VinCodeByte4_enum"
  Data Type Conversion5/1 -> Display6/1  "VINP_VinCodeByte5_enum"
  Data Type Conversion6/1 -> Display7/1  "VINP_VinCodeByte6_enum"
  Demux/8 -> Data Type Conversion7/1
  Demux/9 -> Data Type Conversion8/1
  Demux/10 -> Data Type Conversion9/1
  Demux/11 -> Data Type Conversion10/1
  Demux/12 -> Data Type Conversion11/1
  Demux/13 -> Data Type Conversion12/1
  Demux/14 -> Data Type Conversion13/1
  Demux/15 -> Data Type Conversion14/1
  Demux/16 -> Data Type Conversion15/1
  Demux/17 -> Data Type Conversion16/1
  Data Type Conversion7/1 -> Display8/1  "VINP_VinCodeByte7_enum"
  Data Type Conversion8/1 -> Display9/1  "VINP_VinCodeByte8_enum"
  Data Type Conversion9/1 -> Display10/1  "VINP_VinCodeByte9_enum"
  Data Type Conversion10/1 -> Display11/1  "VINP_VinCodeByte10_enum"
  Data Type Conversion11/1 -> Display12/1  "VINP_VinCodeByte11_enum"
  Data Type Conversion12/1 -> Display13/1  "VINP_VinCodeByte12_enum"
  Data Type Conversion13/1 -> Display14/1  "VINP_VinCodeByte13_enum"
  Data Type Conversion14/1 -> Display15/1  "VINP_VinCodeByte14_enum"
  Data Type Conversion15/1 -> Display16/1  "VINP_VinCodeByte15_enum"
  Data Type Conversion16/1 -> Display17/1  "VINP_VinCodeByte16_enum"

== system SWC_FDC_type/run_SWC_FDC_RxTx_5ms_sys/HALOUT_AFTER/R_E2E_CAN3_VCU1_CSOP_Write_CAN3_VCU1 ==
  Enable : EnablePort
  R_E2E_CAN3_VCU1_CSOP_Write_CAN3_VCU1 : FunctionCaller  FunctionPrototype=R_E2E_CAN3_VCU1_CSOP_Write_CAN3_VCU1()

== system SWC_FDC_type/run_SWC_FDC_RxTx_5ms_sys/HALOUT_AFTER/R_E2E_CAN3_VCU1_toNIDEC_CSOP_Write_CAN3_VCU1_toNIDEC ==
  In1 : EnablePort
  R_E2E_CAN3_VCU1_toNIDEC_CSOP_Write_CAN3_VCU1_toNIDEC : FunctionCaller  FunctionPrototype=R_E2E_CAN3_VCU1_toNIDEC_CSOP_Write_CAN3_VCU1_toNIDEC()

== system SWC_FDC_type/run_SWC_FDC_RxTx_5ms_sys/HALOUT_AFTER/R_E2E_CAN4_VCU1_CSOP_Write_CAN4_VCU1 ==
  In1 : EnablePort
  R_E2E_CAN4_VCU1_CSOP_Write_CAN4_VCU1 : FunctionCaller  FunctionPrototype=R_E2E_CAN4_VCU1_CSOP_Write_CAN4_VCU1()

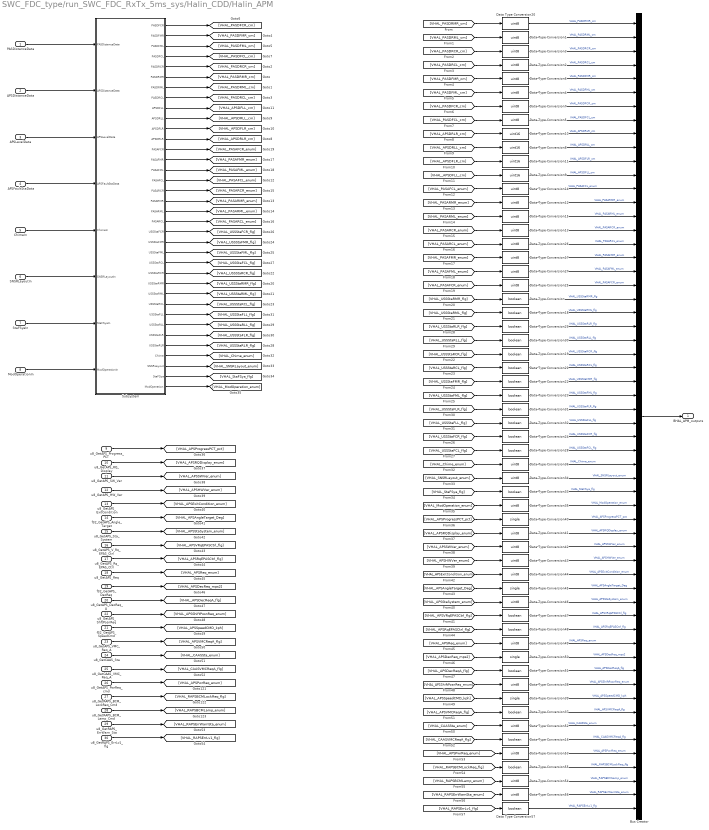
== system SWC_FDC_type/run_SWC_FDC_RxTx_5ms_sys/Halin_CDD/Halin_APM ==
  PASDistanceData : Inport
  APSDistanceData : Inport  Port=2
  APSLevelData : Inport  Port=3
  APSFaultStaData : Inport  Port=4
  ChimeIn : Inport  Port=5
  SNSRLayoutIn : Inport  Port=6
  StaFSyaIn : Inport  Port=7
  ModOperationIn : Inport  Port=8
  u8_GetAPS_Progress_PCT : Inport  Port=9
  u8_GetAPS_RQ_Display : Inport  Port=10
  u8_GetAPS_SW_Ver : Inport  Port=11
  u8_GetAPS_HW_Ver : Inport  Port=12
  u8_GetAPS_ExitCondition : Inport  Port=13
  f32_GetAPS_Angle_Target : Inport  Port=14
  u8_GetAPS_Sta_System : Inport  Port=15
  u8_GetAPS_V_Rq_EPAS_Ctrl : Inport  Port=16
  u8_GetAPS_Rq_EPAS_Ctrl : Inport  Port=17
  u8_GetAPS_Req : Inport  Port=18
  f32_GetAPS_DecReq : Inport  Port=19
  u8_GetAPS_DecReq_A : Inport  Port=20
  f32_GetAPS_SpeedCmd : Inport  Port=21
  u8_GetAPS_ShftPosnReq : Inport  Port=22
  u8_GetAPS_VMC_Req_A : Inport  Port=23
  u8_GetCAAS_Sta : Inport  Port=24
  u8_GetCAAS_VMC_Req_A : Inport  Port=25
  u8_GetAPS_PwrReq_cmd : Inport  Port=26
  u8_GetRAPS_BCM_LockReq_Cmd : Inport  Port=27
  u8_GetRAPS_BCM_Lamp_Cmd : Inport  Port=28
  u8_GetRAPS_ErrWarn_Sta : Inport  Port=29
  u8_GetRAPS_ErrLv1_flg : Inport  Port=30
  Bus Creator : BusCreator  Inputs=58
  Data Type Conversion{,16,18..19,21..24,28..33,37,47..48,51,55,57} (20 alike) : DataTypeConversion  OutDataTypeStr=boolean
  Data Type Conversion{1..7,12..15,17,20,25..27,34..36,38,41..44,46,49,52..54,56} (30 alike) : DataTypeConversion  OutDataTypeStr=uint8
  Data Type Conversion{8..11} (4 alike) : DataTypeConversion  OutDataTypeStr=uint16
  Data Type Conversion{39..40,45,50} (4 alike) : DataTypeConversion  OutDataTypeStr=single
  Subsystem : Subsystem
  BHAL_APM_outputs : Outport
  wires:
  [VHAL_USSStaRMR_flg] -> Data Type Conversion/1
  Data Type Conversion4/1 -> Bus Creator/6  "VHAL_PASDFML_cm"
  Subsystem/11(APSDFLR) -> [VHAL_APSDFLR_cm]
  [VHAL_PASARCL_enum] -> Data Type Conversion26/1
  Subsystem/36(ModOperation) -> [VHAL_ModOperation_enum]
  Bus Creator/1 -> BHAL_APM_outputs/1
  [VHAL_PASDRCR_cm] -> Data Type Conversion3/1
  [VHAL_PASDRML_cm] -> Data Type Conversion1/1
  Data Type Conversion15/1 -> Bus Creator/15  "VHAL_PASARML_enum"
  [VHAL_USSStaFCR_flg] -> Data Type Conversion24/1
  [VHAL_SNSRLayout_enum] -> Data Type Conversion34/1
  Subsystem/12(APSDRLR) -> [VHAL_APSDRLR_cm]
  Data Type Conversion3/1 -> Bus Creator/3  "VHAL_PASDRCR_cm"
  [VHAL_APSDRLR_cm] -> Data Type Conversion10/1
  Data Type Conversion12/1 -> Bus Creator/14  "VHAL_PASARMR_enum"
  Data Type Conversion33/1 -> Bus Creator/35  "VHAL_StaFSya_flg"
  [VHAL_PASARCR_enum] -> Data Type Conversion13/1
  Subsystem/9(APSDFLL) -> [VHAL_APSDFLL_cm]
  [VHAL_StaFSya_flg] -> Data Type Conversion33/1
  [VHAL_USSStaRLL_flg] -> Data Type Conversion30/1
  Subsystem/4(PASDFCL) -> [VHAL_PASDFCL_cm]
  Subsystem/35(StaFSya) -> [VHAL_StaFSya_flg]
  Subsystem/20(PASARCL) -> [VHAL_PASARCL_enum]
  [VHAL_PASDFML_cm] -> Data Type Conversion4/1
  [VHAL_PASDRMR_cm] -> Data Type Conversion20/1
  Subsystem/16(PASAFCL) -> [VHAL_PASAFCL_enum]
  [VHAL_USSStaFCL_flg] -> Data Type Conversion28/1
  Subsystem/18(PASARMR) -> [VHAL_PASARMR_enum]
  Data Type Conversion13/1 -> Bus Creator/16  "VHAL_PASARCR_enum"
  [VHAL_PASARML_enum] -> Data Type Conversion15/1
  [VHAL_APSDFLL_cm] -> Data Type Conversion9/1
  Subsystem/15(PASAFML) -> [VHAL_PASAFML_enum]
  [VHAL_USSStaFLL_flg] -> Data Type Conversion32/1
  Subsystem/8(PASDRCL) -> [VHAL_PASDRCL_cm]
  Subsystem/27(USSStaRML) -> [VHAL_USSStaRML_flg]
  Data Type Conversion6/1 -> Bus Creator/5  "VHAL_PASDFMR_cm"
  [VHAL_PASAFMR_enum] -> Data Type Conversion17/1
  Data Type Conversion28/1 -> Bus Creator/32  "VHAL_USSStaFCL_flg"
  Subsystem/3(PASDFML) -> [VHAL_PASDFML_cm]
  Data Type Conversion9/1 -> Bus Creator/12  "VHAL_APSDFLL_cm"
  Subsystem/24(USSStaFCL) -> [VHAL_USSStaFCL_flg]
  [VHAL_PASAFCL_enum] -> Data Type Conversion14/1
  [VHAL_USSStaFLR_flg] -> Data Type Conversion31/1
  Subsystem/34(SNSRLayout) -> [VHAL_SNSRLayout_enum]
  Subsystem/29(USSStaFLL) -> [VHAL_USSStaFLL_flg]
  Subsystem/21(USSStaFCR) -> [VHAL_USSStaFCR_flg]
  [VHAL_PASDRCL_cm] -> Data Type Conversion2/1
  Data Type Conversion14/1 -> Bus Creator/13  "VHAL_PASAFCL_enum"
  Subsystem/1(PASDFCR) -> [VHAL_PASDFCR_cm]
  Data Type Conversion7/1 -> Bus Creator/7  "VHAL_PASDFCR_cm"
  Subsystem/2(PASDFMR) -> [VHAL_PASDFMR_cm]
  Subsystem/30(USSStaRLL) -> [VHAL_USSStaRLL_flg]
  Data Type Conversion17/1 -> Bus Creator/18  "VHAL_PASAFMR_enum"
  [VHAL_PASARMR_enum] -> Data Type Conversion12/1
  Data Type Conversion32/1 -> Bus Creator/30  "VHAL_USSStaFLL_flg"
  Subsystem/7(PASDRML) -> [VHAL_PASDRML_cm]
  Subsystem/26(USSStaRMR) -> [VHAL_USSStaRMR_flg]
  Data Type Conversion20/1 -> Bus Creator/1  "VHAL_PASDRMR_cm"
  [VHAL_USSStaRCL_flg] -> Data Type Conversion21/1
  Subsystem/10(APSDRLL) -> [VHAL_APSDRLL_cm]
  Data Type Conversion34/1 -> Bus Creator/34  "VHAL_SNSRLayout_enum"
  [VHAL_Chime_enum] -> Data Type Conversion36/1
  Data Type Conversion18/1 -> Bus Creator/22  "VHAL_USSStaRML_flg"
  [VHAL_PASDFMR_cm] -> Data Type Conversion6/1
  Data Type Conversion31/1 -> Bus Creator/29  "VHAL_USSStaFLR_flg"
  Data Type Conversion10/1 -> Bus Creator/9  "VHAL_APSDRLR_cm"
  Data Type Conversion35/1 -> Bus Creator/36  "VHAL_ModOperation_enum"
  Subsystem/31(USSStaFLR) -> [VHAL_USSStaFLR_flg]
  Data Type Conversion8/1 -> Bus Creator/10  "VHAL_APSDRLL_cm"
  [VHAL_USSStaRML_flg] -> Data Type Conversion18/1
  Subsystem/19(PASARML) -> [VHAL_PASARML_enum]
  [VHAL_USSStaFMR_flg] -> Data Type Conversion22/1
  Subsystem/22(USSStaFMR) -> [VHAL_USSStaFMR_flg]
  Data Type Conversion25/1 -> Bus Creator/20  "VHAL_PASAFCR_enum"
  Subsystem/33(Chime) -> [VHAL_Chime_enum]
  Data Type Conversion11/1 -> Bus Creator/11  "VHAL_APSDFLR_cm"
  Data Type Conversion36/1 -> Bus Creator/33  "VHAL_Chime_enum"
  [VHAL_APSDFLR_cm] -> Data Type Conversion11/1
  Subsystem/13(PASAFCR) -> [VHAL_PASAFCR_enum]
  [VHAL_PASDFCL_cm] -> Data Type Conversion5/1
  Data Type Conversion/1 -> Bus Creator/21  "VHAL_USSStaRMR_flg"
  Data Type Conversion2/1 -> Bus Creator/4  "VHAL_PASDRCL_cm"
  [VHAL_USSStaFML_flg] -> Data Type Conversion23/1
  Data Type Conversion1/1 -> Bus Creator/2  "VHAL_PASDRML_cm"
  [VHAL_USSStaRCR_flg] -> Data Type Conversion19/1
  Subsystem/25(USSStaRCR) -> [VHAL_USSStaRCR_flg]
  Subsystem/28(USSStaRCL) -> [VHAL_USSStaRCL_flg]
  [VHAL_ModOperation_enum] -> Data Type Conversion35/1
  Data Type Conversion19/1 -> Bus Creator/25  "VHAL_USSStaRCR_flg"
  Subsystem/5(PASDRCR) -> [VHAL_PASDRCR_cm]
  Data Type Conversion26/1 -> Bus Creator/17  "VHAL_PASARCL_enum"
  Data Type Conversion27/1 -> Bus Creator/19  "VHAL_PASAFML_enum"
  Subsystem/23(USSStaFML) -> [VHAL_USSStaFML_flg]
  Subsystem/17(PASARCR) -> [VHAL_PASARCR_enum]
  [VHAL_APSDRLL_cm] -> Data Type Conversion8/1
  Subsystem/6(PASDRMR) -> [VHAL_PASDRMR_cm]
  Data Type Conversion21/1 -> Bus Creator/26  "VHAL_USSStaRCL_flg"
  Data Type Conversion24/1 -> Bus Creator/31  "VHAL_USSStaFCR_flg"
  Data Type Conversion23/1 -> Bus Creator/28  "VHAL_USSStaFML_flg"
  Data Type Conversion5/1 -> Bus Creator/8  "VHAL_PASDFCL_cm"
  [VHAL_PASAFCR_enum] -> Data Type Conversion25/1
  [VHAL_PASDFCR_cm] -> Data Type Conversion7/1
  Data Type Conversion29/1 -> Bus Creator/23  "VHAL_USSStaRLR_flg"
  [VHAL_USSStaRLR_flg] -> Data Type Conversion29/1
  Subsystem/14(PASAFMR) -> [VHAL_PASAFMR_enum]
  Data Type Conversion30/1 -> Bus Creator/24  "VHAL_USSStaRLL_flg"
  Subsystem/32(USSStaRLR) -> [VHAL_USSStaRLR_flg]
  [VHAL_PASAFML_enum] -> Data Type Conversion27/1
  Data Type Conversion22/1 -> Bus Creator/27  "VHAL_USSStaFMR_flg"
  APSDistanceData/1 -> Subsystem/2(APSDistanceData)
  APSFaultStaData/1 -> Subsystem/4(APSFaultStaData)
  APSLevelData/1 -> Subsystem/3(APSLevelData)
  ChimeIn/1 -> Subsystem/5(ChimeIn)
  SNSRLayoutIn/1 -> Subsystem/6(SNSRLayoutIn)
  StaFSyaIn/1 -> Subsystem/7(StaFSyaIn)
  ModOperationIn/1 -> Subsystem/8(ModOperationIn)
  PASDistanceData/1 -> Subsystem/1(PASDistanceData)
  u8_GetAPS_HW_Ver/1 -> [VHAL_APSHWVer_enum]
  u8_GetAPS_Progress_PCT/1 -> [VHAL_APSProgressPCT_pct]
  u8_GetAPS_Req/1 -> [VHAL_APSReq_enum]
  u8_GetAPS_Sta_System/1 -> [VHAL_APSStaSystem_enum]
  u8_GetAPS_SW_Ver/1 -> [VHAL_APSSWVer_enum]
  u8_GetAPS_V_Rq_EPAS_Ctrl/1 -> [VHAL_APSVRqEPASCtrl_flg]
  u8_GetAPS_ExitCondition/1 -> [VHAL_APSExitCondition_enum]
  u8_GetCAAS_Sta/1 -> [VHAL_CAASSta_enum]
  u8_GetAPS_VMC_Req_A/1 -> [VHAL_APSVMCReqA_flg]
  f32_GetAPS_SpeedCmd/1 -> [VHAL_APSSpeedCMD_kph]
  u8_GetAPS_Rq_EPAS_Ctrl/1 -> [VHAL_APSRqEPASCtrl_flg]
  u8_GetAPS_ShftPosnReq/1 -> [VHAL_APSShiftPosnReq_enum]
  u8_GetAPS_DecReq_A/1 -> [VHAL_APSDecReqA_flg]
  f32_GetAPS_Angle_Target/1 -> [VHAL_APSAngleTarget_Deg]
  u8_GetAPS_RQ_Display/1 -> [VHAL_APSRQDisplay_enum]
  f32_GetAPS_DecReq/1 -> [VHAL_APSDecReq_mps2]
  u8_GetCAAS_VMC_Req_A/1 -> [VHAL_CAASVMCReqA_flg]
  Data Type Conversion47/1 -> Bus Creator/44  "VHAL_APSVRqEPASCtrl_flg"
  Data Type Conversion50/1 -> Bus Creator/47  "VHAL_APSDecReq_mps2"
  Data Type Conversion39/1 -> Bus Creator/50  "VHAL_APSSpeedCMD_kph"
  Data Type Conversion43/1 -> Bus Creator/40  "VHAL_APSHWVer_enum"
  Data Type Conversion38/1 -> Bus Creator/49  "VHAL_APSShiftPosnReq_enum"
  Data Type Conversion42/1 -> Bus Creator/39  "VHAL_APSSWVer_enum"
  [VHAL_APSVRqEPASCtrl_flg] -> Data Type Conversion47/1
  Data Type Conversion51/1 -> Bus Creator/48  "VHAL_APSDecReqA_flg"
  Data Type Conversion46/1 -> Bus Creator/43  "VHAL_APSStaSystem_enum"
  Data Type Conversion44/1 -> Bus Creator/41  "VHAL_APSExitCondition_enum"
  [VHAL_APSVMCReqA_flg] -> Data Type Conversion37/1
  [VHAL_APSReq_enum] -> Data Type Conversion49/1
  [VHAL_APSSpeedCMD_kph] -> Data Type Conversion39/1
  Data Type Conversion48/1 -> Bus Creator/45  "VHAL_APSRqEPASCtrl_flg"
  [VHAL_APSShiftPosnReq_enum] -> Data Type Conversion38/1
  Data Type Conversion52/1 -> Bus Creator/52  "VHAL_CAASSta_enum"
  Data Type Conversion45/1 -> Bus Creator/42  "VHAL_APSAngleTarget_Deg"
  Data Type Conversion49/1 -> Bus Creator/46  "VHAL_APSReq_enum"
  [VHAL_CAASSta_enum] -> Data Type Conversion52/1
  [VHAL_APSRqEPASCtrl_flg] -> Data Type Conversion48/1
  [VHAL_APSStaSystem_enum] -> Data Type Conversion46/1
  Data Type Conversion40/1 -> Bus Creator/37  "VHAL_APSProgressPCT_pct"
  [VHAL_APSExitCondition_enum] -> Data Type Conversion44/1
  [VHAL_APSSWVer_enum] -> Data Type Conversion42/1
  [VHAL_APSHWVer_enum] -> Data Type Conversion43/1
  [VHAL_APSAngleTarget_Deg] -> Data Type Conversion45/1
  [VHAL_APSDecReq_mps2] -> Data Type Conversion50/1
  [VHAL_APSProgressPCT_pct] -> Data Type Conversion40/1
  [VHAL_APSDecReqA_flg] -> Data Type Conversion51/1
  [VHAL_APSRQDisplay_enum] -> Data Type Conversion41/1
  Data Type Conversion41/1 -> Bus Creator/38  "VHAL_APSRQDisplay_enum"
  Data Type Conversion37/1 -> Bus Creator/51  "VHAL_APSVMCReqA_flg"
  [VHAL_CAASVMCReqA_flg] -> Data Type Conversion16/1
  Data Type Conversion16/1 -> Bus Creator/53  "VHAL_CAASVMCReqA_flg"
  u8_GetRAPS_BCM_LockReq_Cmd/1 -> [VHAL_RAPSBCMLockReq_flg]
  u8_GetRAPS_BCM_Lamp_Cmd/1 -> [VHAL_RAPSBCMLamp_enum]
  u8_GetAPS_PwrReq_cmd/1 -> [VHAL_APSPwrReq_enum]
  u8_GetRAPS_ErrWarn_Sta/1 -> [VHAL_RAPSErrWarnSta_enum]
  u8_GetRAPS_ErrLv1_flg/1 -> [VHAL_RAPSErrLv1_flg]
  [VHAL_APSPwrReq_enum] -> Data Type Conversion53/1
  [VHAL_RAPSBCMLockReq_flg] -> Data Type Conversion55/1
  [VHAL_RAPSBCMLamp_enum] -> Data Type Conversion54/1
  Data Type Conversion54/1 -> Bus Creator/56  "VHAL_RAPSBCMLamp_enum"
  Data Type Conversion55/1 -> Bus Creator/55  "VHAL_RAPSBCMLockReq_flg"
  Data Type Conversion53/1 -> Bus Creator/54  "VHAL_APSPwrReq_enum"
  [VHAL_RAPSErrWarnSta_enum] -> Data Type Conversion56/1
  [VHAL_RAPSErrLv1_flg] -> Data Type Conversion57/1
  Data Type Conversion57/1 -> Bus Creator/58  "VHAL_RAPSErrLv1_flg"
  Data Type Conversion56/1 -> Bus Creator/57  "VHAL_RAPSErrWarnSta_enum"
